simulink model "test_ventilation"  (Simulink 8.2)
settings: Solver=VariableStepDiscrete  StartTime=0.0  StopTime=365*24*3600  RelTol=1e-3
libraries: carnot x3
settings Model: Creator=drhf  LastModifiedBy=drhf

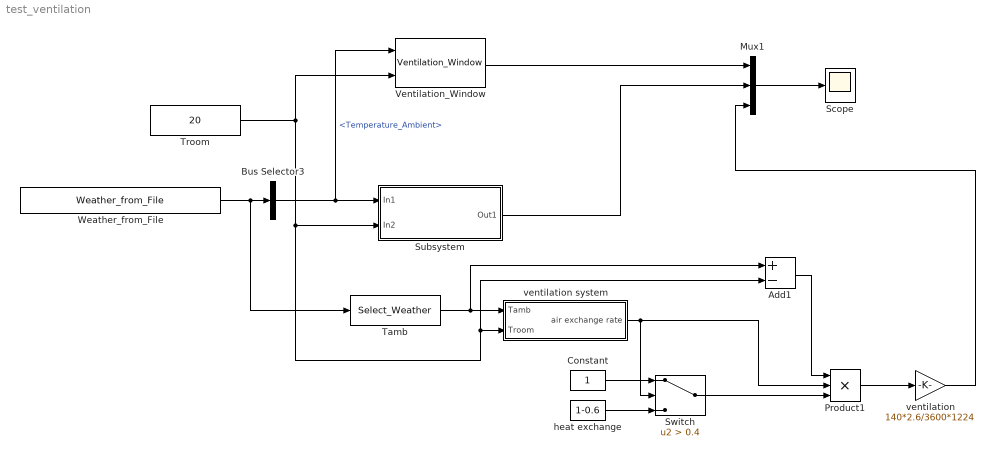
== system test_ventilation ==
  Add1 : Sum  Inputs=+-
  Bus Selector3 : BusSelector  OutputSignals=Temperature_Ambient
  Constant : Constant
  Mux1 : Mux  Inputs=3
  Product1 : Product  Inputs=3
  Scope : Scope
      settings: TickLabels=on  YMin=-7.5  YMax=35  SampleTime=3600*3
  Subsystem : Subsystem  mask{Ahabit=140, Hroom=2.6, vent=0.4, rec=0.6}
      mask prompts: Ahabit "Surface"; Hroom "Height of room"; vent "Ventilation"; rec "Heat recovery"
  Switch : Switch  Criteria=u2 > Threshold  Threshold=0.4
  Tamb : carnot/Weather/Select_Weather  v=6
  Troom : Constant  Value=20
  Ventilation_Window : carnot/Source/Ventilation/Ventilation_Window  vent=0.4  rec=0.6  Vhouse=140*2.6
  Weather_from_File : carnot/Weather/Weather_from_File  file=DE_TRY2010_12_averageYear  ext=.mat
  heat exchange : Constant  Value=1-0.6
  ventilation : Gain  Gain=140*2.6/3600*1224
  ventilation system : Subsystem
  wires:
  Troom/1 -> Subsystem/2(In2), ventilation system/2(Troom), Add1/2, Ventilation_Window/2
  Weather_from_File/1 -> Bus Selector3/1, Tamb/1
  Bus Selector3/1 -> Subsystem/1(In1), Ventilation_Window/1  "<Temperature_Ambient>"
  Ventilation_Window/1 -> Mux1/1
  Mux1/1 -> Scope/1
  Subsystem/1(Out1) -> Mux1/2
  Add1/1 -> Product1/1
  Tamb/1 -> ventilation system/1(Tamb), Add1/1
  ventilation system/1(air exchange rate) -> Switch/2, Product1/2
  Switch/1 -> Product1/3
  heat exchange/1 -> Switch/3
  Constant/1 -> Switch/1
  Product1/1 -> ventilation/1
  ventilation/1 -> Mux1/3

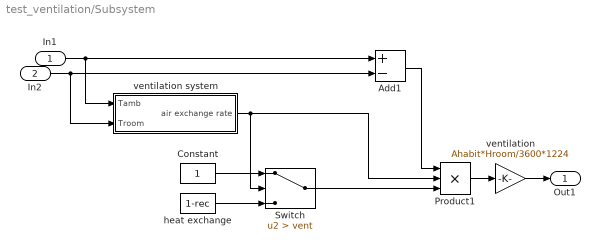
== system test_ventilation/Subsystem ==
  In1 : Inport
  In2 : Inport  Port=2
  Add1 : Sum  Inputs=+-
  Constant : Constant
  Product1 : Product  Inputs=3
  Switch : Switch  Criteria=u2 > Threshold  Threshold=vent
  heat exchange : Constant  Value=1-rec
  ventilation : Gain  Gain=Ahabit*Hroom/3600*1224
  ventilation system : Subsystem
  Out1 : Outport
  wires:
  Product1/1 -> ventilation/1
  Add1/1 -> Product1/1
  ventilation system/1(air exchange rate) -> Switch/2, Product1/2
  Switch/1 -> Product1/3
  Constant/1 -> Switch/1
  heat exchange/1 -> Switch/3
  In1/1 -> Add1/1, ventilation system/1(Tamb)
  In2/1 -> Add1/2, ventilation system/2(Troom)
  ventilation/1 -> Out1/1

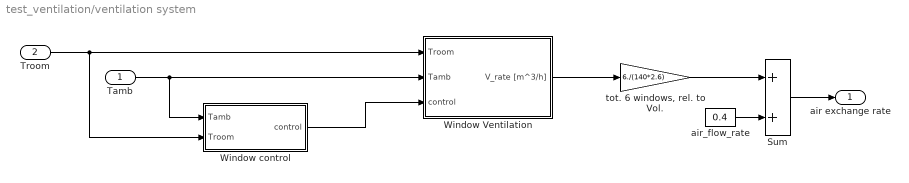
== system test_ventilation/ventilation system ==
  Tamb : Inport
  Troom : Inport  Port=2
  Sum : Sum
  Window Ventilation : Subsystem  mask(window ventilation){alpha=10, H=1, W=1}
      mask prompts: alpha "maximal opening angle (°)"; H "height of window (m)"; W "width of window (m)"
      mask help: Simulates the free driven ventilation through a window with an opening angle of [0,1]* max. angle. Valid for angles between 8° and 180°. Output is the VOLUME FLOW RATE in m^3/h. Calculation based on the Ansatz from Weber.
      mask Display: plot(0,10,90,80,[20 70 70 20 20],[20 20 70 70 20],[20 70 80 30 20],[20 20 65 65 20])
  Window control : Subsystem
  air_flow_rate : Constant  Value=0.4
  "tot. 6 windows, rel. to Vol." : Gain  Gain=6./(140*2.6)
  air exchange rate : Outport
  wires:
  Window control/1(control) -> Window Ventilation/3(control)
  Window Ventilation/1(V_rate [m^3/h]) -> "tot. 6 windows, rel. to Vol."/1
  air_flow_rate/1 -> Sum/2
  Sum/1 -> air exchange rate/1
  "tot. 6 windows, rel. to Vol."/1 -> Sum/1
  Troom/1 -> Window Ventilation/1(Troom), Window control/2(Troom)
  Tamb/1 -> Window control/1(Tamb), Window Ventilation/2(Tamb)

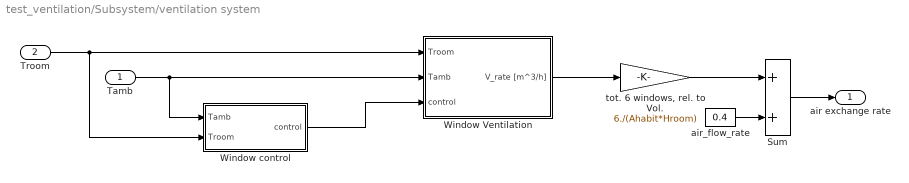
== system test_ventilation/Subsystem/ventilation system ==
  Tamb : Inport
  Troom : Inport  Port=2
  Sum : Sum
  Window Ventilation : Subsystem  mask(window ventilation){alpha=10, H=1, W=1}
      mask prompts: alpha "maximal opening angle (°)"; H "height of window (m)"; W "width of window (m)"
      mask help: Simulates the free driven ventilation through a window with an opening angle of [0,1]* max. angle. Valid for angles between 8° and 180°. Output is the VOLUME FLOW RATE in m^3/h. Calculation based on the Ansatz from Weber.
      mask Display: plot(0,10,90,80,[20 70 70 20 20],[20 20 70 70 20],[20 70 80 30 20],[20 20 65 65 20])
  Window control : Subsystem
  air_flow_rate : Constant  Value=0.4
  "tot. 6 windows, rel. to Vol." : Gain  Gain=6./(Ahabit*Hroom)
  air exchange rate : Outport
  wires:
  Window control/1(control) -> Window Ventilation/3(control)
  Window Ventilation/1(V_rate [m^3/h]) -> "tot. 6 windows, rel. to Vol."/1
  air_flow_rate/1 -> Sum/2
  Sum/1 -> air exchange rate/1
  "tot. 6 windows, rel. to Vol."/1 -> Sum/1
  Troom/1 -> Window Ventilation/1(Troom), Window control/2(Troom)
  Tamb/1 -> Window control/1(Tamb), Window Ventilation/2(Tamb)

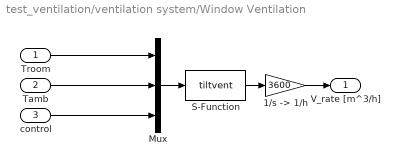
== system test_ventilation/ventilation system/Window Ventilation ==
  Troom : Inport
  Tamb : Inport  Port=2
  control : Inport  Port=3
  "1/s -> 1/h" : Gain  Gain=3600
  Mux : Mux  Inputs=3
  S-Function : S-Function  FunctionName=tiltvent  Parameters=alpha, H, W  EnableBusSupport=off
  V_rate [m^3/h] : Outport
  wires:
  Tamb/1 -> Mux/2
  control/1 -> Mux/3
  S-Function/1 -> "1/s -> 1/h"/1
  Mux/1 -> S-Function/1
  Troom/1 -> Mux/1
  "1/s -> 1/h"/1 -> V_rate [m^3/h]/1

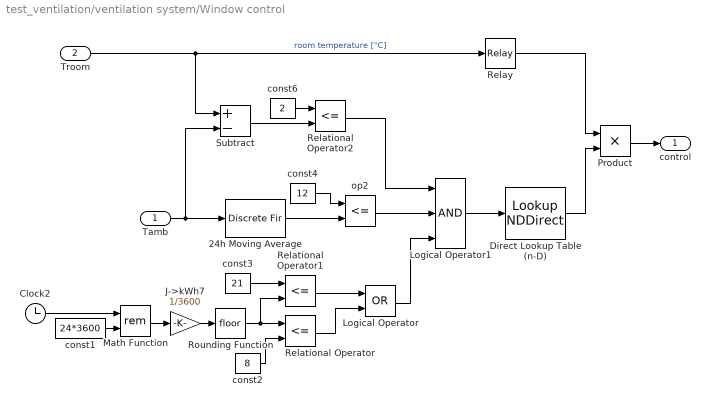
== system test_ventilation/ventilation system/Window control ==
  Tamb : Inport
  Troom : Inport  Port=2
  24h Moving Average : DiscreteFir  Coefficients=ones(1,24)*(1/24)  SampleTime=3600  AccumDataTypeStr=Inherit: Same as product output  RndMeth=Nearest
  Clock2 : Clock
  Direct Lookup Table (n-D) : LookupNDDirect  NumberOfTableDimensions=1  Table=[0 1]
  J->kWh7 : Gain  Gain=1/3600  SaturateOnIntegerOverflow=on  OutDataTypeStr=Inherit: Same as input  ParamDataTypeStr=Inherit: Same as input
  Logical Operator : Logic  Operator=OR  AllPortsSameDT=off  OutDataTypeStr=boolean
  Logical Operator1 : Logic  Inputs=3  AllPortsSameDT=off  OutDataTypeStr=boolean
  Math Function : Math  Operator=rem  SaturateOnIntegerOverflow=on
  Product : Product  RndMeth=Zero
  Relational Operator : RelationalOperator  Operator=<=  OutDataTypeStr=boolean
  Relational Operator1 : RelationalOperator  Operator=<=  OutDataTypeStr=boolean
  Relational Operator2 : RelationalOperator  Operator=<=  OutDataTypeStr=boolean
  Relay : Relay  OnSwitchValue=24  OffSwitchValue=23
  Rounding Function : Rounding
  Subtract : Sum  Inputs=+-
  const1 : Constant  Value=24*3600
  const2 : Constant  Value=8
  const3 : Constant  Value=21
  const4 : Constant  Value=12
  const6 : Constant  Value=2
  op2 : RelationalOperator  Operator=<=  OutDataTypeStr=boolean
  control : Outport
  wires:
  Clock2/1 -> Math Function/1
  const1/1 -> Math Function/2
  Math Function/1 -> J->kWh7/1
  J->kWh7/1 -> Rounding Function/1
  Rounding Function/1 -> Relational Operator/1, Relational Operator1/2
  const2/1 -> Relational Operator/2
  const3/1 -> Relational Operator1/1
  Relational Operator1/1 -> Logical Operator/1
  Relational Operator/1 -> Logical Operator/2
  Tamb/1 -> Subtract/2, 24h Moving Average/1
  const4/1 -> op2/1
  Logical Operator/1 -> Logical Operator1/3
  Troom/1 -> Relay/1, Subtract/1  "room temperature [°C]"
  const6/1 -> Relational Operator2/1
  Subtract/1 -> Relational Operator2/2
  Relational Operator2/1 -> Logical Operator1/1
  Logical Operator1/1 -> Direct Lookup Table (n-D)/1
  op2/1 -> Logical Operator1/2
  Direct Lookup Table (n-D)/1 -> Product/2
  Product/1 -> control/1
  Relay/1 -> Product/1
  24h Moving Average/1 -> op2/2

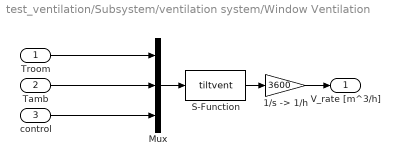
== system test_ventilation/Subsystem/ventilation system/Window Ventilation ==
  Troom : Inport
  Tamb : Inport  Port=2
  control : Inport  Port=3
  "1/s -> 1/h" : Gain  Gain=3600
  Mux : Mux  Inputs=3
  S-Function : S-Function  FunctionName=tiltvent  Parameters=alpha, H, W  EnableBusSupport=off
  V_rate [m^3/h] : Outport
  wires:
  Tamb/1 -> Mux/2
  control/1 -> Mux/3
  S-Function/1 -> "1/s -> 1/h"/1
  Mux/1 -> S-Function/1
  Troom/1 -> Mux/1
  "1/s -> 1/h"/1 -> V_rate [m^3/h]/1

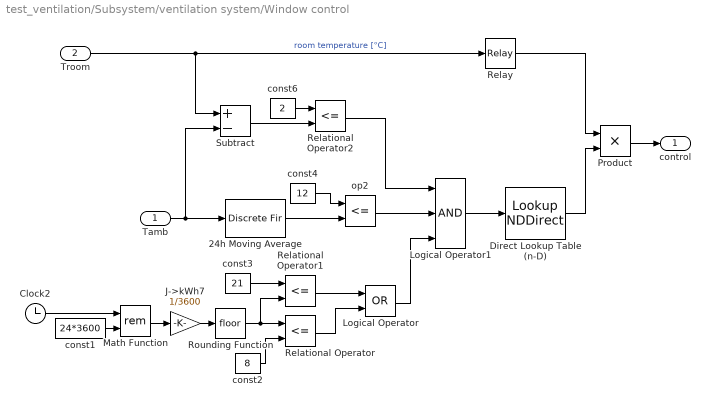
== system test_ventilation/Subsystem/ventilation system/Window control ==
  Tamb : Inport
  Troom : Inport  Port=2
  24h Moving Average : DiscreteFir  Coefficients=ones(1,24)*(1/24)  SampleTime=3600  AccumDataTypeStr=Inherit: Same as product output  RndMeth=Nearest
  Clock2 : Clock
  Direct Lookup Table (n-D) : LookupNDDirect  NumberOfTableDimensions=1  Table=[0 1]
  J->kWh7 : Gain  Gain=1/3600  SaturateOnIntegerOverflow=on  OutDataTypeStr=Inherit: Same as input  ParamDataTypeStr=Inherit: Same as input
  Logical Operator : Logic  Operator=OR  AllPortsSameDT=off  OutDataTypeStr=boolean
  Logical Operator1 : Logic  Inputs=3  AllPortsSameDT=off  OutDataTypeStr=boolean
  Math Function : Math  Operator=rem  SaturateOnIntegerOverflow=on
  Product : Product  RndMeth=Zero
  Relational Operator : RelationalOperator  Operator=<=  OutDataTypeStr=boolean
  Relational Operator1 : RelationalOperator  Operator=<=  OutDataTypeStr=boolean
  Relational Operator2 : RelationalOperator  Operator=<=  OutDataTypeStr=boolean
  Relay : Relay  OnSwitchValue=24  OffSwitchValue=23
  Rounding Function : Rounding
  Subtract : Sum  Inputs=+-
  const1 : Constant  Value=24*3600
  const2 : Constant  Value=8
  const3 : Constant  Value=21
  const4 : Constant  Value=12
  const6 : Constant  Value=2
  op2 : RelationalOperator  Operator=<=  OutDataTypeStr=boolean
  control : Outport
  wires:
  Clock2/1 -> Math Function/1
  const1/1 -> Math Function/2
  Math Function/1 -> J->kWh7/1
  J->kWh7/1 -> Rounding Function/1
  Rounding Function/1 -> Relational Operator/1, Relational Operator1/2
  const2/1 -> Relational Operator/2
  const3/1 -> Relational Operator1/1
  Relational Operator1/1 -> Logical Operator/1
  Relational Operator/1 -> Logical Operator/2
  Tamb/1 -> Subtract/2, 24h Moving Average/1
  const4/1 -> op2/1
  Logical Operator/1 -> Logical Operator1/3
  Troom/1 -> Relay/1, Subtract/1  "room temperature [°C]"
  const6/1 -> Relational Operator2/1
  Subtract/1 -> Relational Operator2/2
  Relational Operator2/1 -> Logical Operator1/1
  Logical Operator1/1 -> Direct Lookup Table (n-D)/1
  op2/1 -> Logical Operator1/2
  Direct Lookup Table (n-D)/1 -> Product/2
  Product/1 -> control/1
  Relay/1 -> Product/1
  24h Moving Average/1 -> op2/2
